simulink model "doc_qam_scatter"  (R2014a)
settings: Solver=ode45  StartTime=0.0  StopTime=250  RelTol=1e-3
undefined symbols (not defined in the file or in its folder): commblksprivate, Info
libraries: commchan3 x1, commrandsrc2 x1, commdigbbndam3 x1
settings Model: ExtModeAutoUpdateStatusClock=off  Creator=The MathWorks Inc.
settings DataIOCC: SignalLoggingSaveFormat=ModelDataLogs  SignalLoggingName=sigsOut
settings OptimizationCC: BlockReduction=off  BooleanDataType=off  ExpressionDepthLimit=2147483647  InitFltsAndDblsToZero=on
settings DebuggingCC: SaveWithParameterizedLinksMsg=none  UnderspecifiedInitializationDetection=Classic  CheckExecutionContextPreStartOutputMsg=on  CheckExecutionContextRuntimeOutputMsg=on  SignalResolutionControl=TryResolveAllWithWarning  SolverPrmCheckMsg=none  InheritedTsInSrcMsg=none  MultiTaskDSMMsg=warning  MultiTaskCondExecSysMsg=none  FcnCallInpInsideContextMsg=UseLocalSettings  StateNameClashWarn=warning  StrictBusMsg=None
settings HardwareCC: TargetUnknown=on
settings ModelReferenceCC: UpdateModelReferenceTargets=IfOutOfDate
settings RTWCC: IncludeERTFirstTime=on
settings GRTTargetCC: TargetFcnLib=ansi_tfl_tmw.mat  CombineOutputUpdateFcns=off  GRTInterface=on

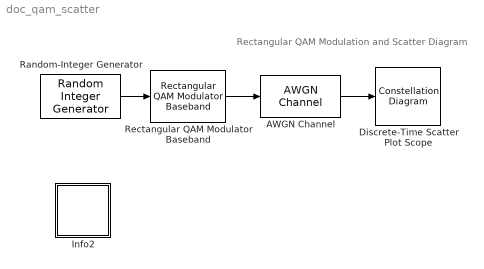
== system doc_qam_scatter ==
  note: Rectangular QAM Modulation and Scatter Diagram
  AWGN Channel : commchan3/AWGN Channel  InputProcessing=Columns as channels (frame based)  seed=1  noiseMode="Signal to noise ratio  (Es/No)"  EbNodB=10  EsNodB=20  SNRdB=10  bitsPerSym=1  Ps=1  Tsym=.1  variance=1
  Discrete-Time Scatter Plot Scope : ConstellationDiagram  Tag=ScatterPlot
  Info2 : Subsystem  AncestorBlock=commblksprivate/Info  mask(Info){}
      settings: OpenFcn=helpview([docroot '/toolbox/comm/comm.map'], 'doc_qam_scatter')
      mask Display: disp('Info')
  Random-Integer Generator : commrandsrc2/Random Integer Generator  mul=16  seed=392  Ts=.1  frameBased=off  sampPerFrame=1  orient=off  outDataType=double
  Rectangular QAM Modulator Baseband : commdigbbndam3/Rectangular QAM Modulator Baseband  M=16  InType=Integer  Enc=Binary  Mapping=[0:15]  PowType=Peak Power  MinDist=2  AvgPow=1  PeakPow=1  Ph=0  outDtype=double  outWordLen=16  outUDDataType=sfix(16)  outFracLenMode=Best precision  outFracLen=15
  wires:
  AWGN Channel/1 -> Discrete-Time Scatter Plot Scope/1
  Random-Integer Generator/1 -> Rectangular QAM Modulator Baseband/1
  Rectangular QAM Modulator Baseband/1 -> AWGN Channel/1

== system doc_qam_scatter/Info2 ==
